simulink model "Dynamic_Wireless_transfer"  (R2024a)
settings: Solver=ode23t  StartTime=0.0  StopTime=10  RelTol=1e-3
undefined symbols (not defined in the file): Ion, Lithium
libraries: spsSeriesRLCBranchLib x6, spsDiodeLib x4, spsIGBTDiodeLib x4, spsCurrentMeasurementLib x3, spsVoltageMeasurementLib x3, spsACVoltageSourceLib x1, spsBatteryLib x1, spsMutualInductanceLib x1, spsPWMGeneratorDCDCLib x1, spsUniversalBridgeLib x1, sps_lib x1
settings Model: Creator=User  LastModifiedBy=User

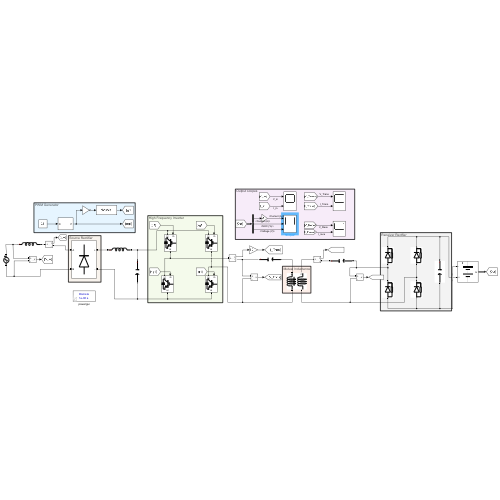
[thumbnail: Simulink's stored preview of the top-level diagram]
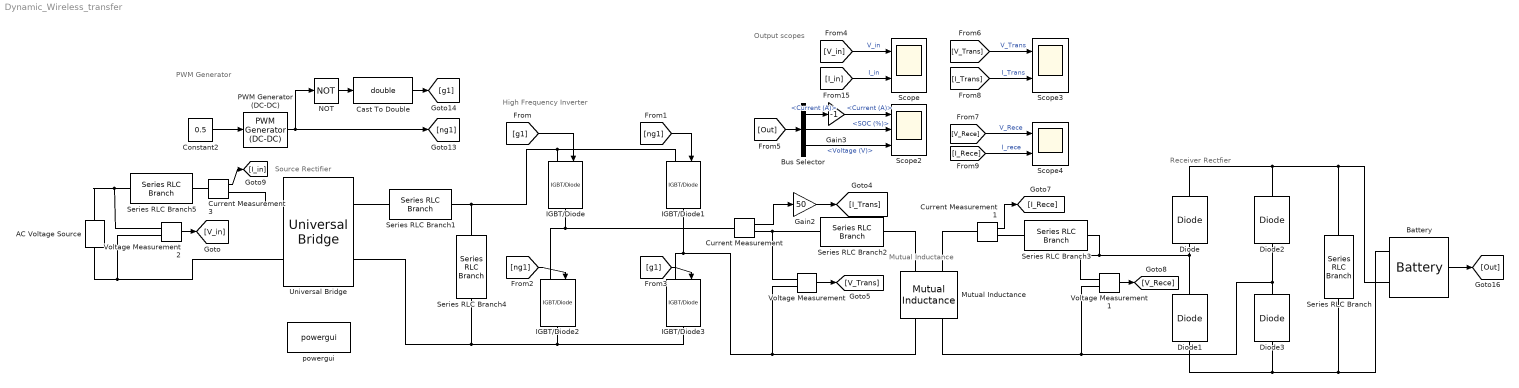
== system Dynamic_Wireless_transfer ==
  note: PWM Generator
  note: Mutual Inductance
  note: Source Rectifier
  note: Output scopes
  note: Receiver Rectfier
  note: High Frequency Inverter
  AC Voltage Source : spsACVoltageSourceLib/AC Voltage Source  Amplitude=500  Phase=180  Frequency=60  SampleTime=0  Measurements=Voltage  BusType=swing  Pref=10e3  Qref=0  Qmin=-inf  Qmax=+inf
  Battery : spsBatteryLib/Battery  BatType=Lithium-Ion  ShowTempParam=off  ThermalPreset=no  ShowAgeParam=off  NomV=360  NomQ=100  SOC=50  Batt_Tr=10  PresetModel=on  MaxQ=100  MinV=270  FullV=419.0354  Dis_rate=43.4783  R=0.036  Normal_OP=90.4348  expZone="[388.9389      4.913043]"  current=[6.5 13 32.5]  Units=Time  Tci=20  NomT=20  T2=-30  MaxQ2=4.8  FullV2=7.1  Normal_OP2=5.655  expZone2="[6.58           1]"  Rca=0.6  ti=2000  Dp=0  Neq0=0  Tsim=1e6  Ta1=25  Qeol=5.4*0.9  Reol=0.013333*1.2  Char_age=[2.3478, 3]  Dis_age=[2.3478, 10]  N1=1500  N2=10500  N3=1000  N4=1400  Ta2=45  N5=950
  Bus Selector : BusSelector  OutputSignals=Current (A),SOC (%),Voltage (V)
  Cast To Double : DataTypeConversion  OutDataTypeStr=double  SaturateOnIntegerOverflow=off  RndMeth=Floor
  Constant2 : Constant  Value=0.5
  Current Measurement : spsCurrentMeasurementLib/Current Measurement  PhasorSimulation=off  OutputType=Complex  PSBequivalent=0
  Current Measurement1 : spsCurrentMeasurementLib/Current Measurement  PhasorSimulation=off  OutputType=Complex  PSBequivalent=0
  Current Measurement3 : spsCurrentMeasurementLib/Current Measurement  PhasorSimulation=off  OutputType=Complex  PSBequivalent=0
  Diode{,1..3} (4 alike) : spsDiodeLib/Diode  Ron=0.001  Lon=0  Vf=0.8  IC=0  UseSnubber=0  Rs=500  Cs=250e-9  Measurements=off
  Gain2 : Gain  Gain=50
  Gain3 : Gain  Gain=-1
  IGBT/Diode{,1..3} (4 alike) : spsIGBTDiodeLib/IGBT//Diode  Ron=1e-3  Rs=1e5  Cs=inf  Measurements=off
  Mutual Inductance : spsMutualInductanceLib/Mutual Inductance  LConnTagsString=a|b  RConnTagsString=A|B  TypeOfMutual=Two or three windings with equal mutual terms  NumberOfWindings=3  SelfImpedance1=[1e-3 266.16e-6]  SelfImpedance2=[1e-3 256.79e-6]  ThreeWindings=off  SelfImpedance3=[ 1.1 1.1e-03]  MutualImpedance=[0 85.46e-6]  InductanceMatrix="[1.0 0.9  0.9 ;  0.9 1.0  0.9;  0.9 0.9 1.0 ] * 1e-3"  ResistanceMatrix="[1.0 0.9  0.9 ;  0.9 1.0  0.9;  0.9 0.9 1.0 ]"  Measurements=None
      settings: LibrarySourceBlock=sps_lib/Passives/Mutual Inductance
  NOT : Logic  Operator=NOT  IconShape=distinctive  AllPortsSameDT=off  OutDataTypeStr=boolean
  PWM Generator (DC-DC) : spsPWMGeneratorDCDCLib/PWM Generator (DC-DC)  Fsw=30000  Ts=0
  Scope : Scope  NumInputPorts=2
  Scope2 : Scope  NumInputPorts=3
  Scope3 : Scope  NumInputPorts=2
  Scope4 : Scope  NumInputPorts=2
  Series RLC Branch : spsSeriesRLCBranchLib/Series RLC Branch  LConnTagsString=__new0  RConnTagsString=__new0  BranchType=C  Resistance=1  Inductance=1e-3  SetiL0=off  InitialCurrent=0  Capacitance=300e-6  Setx0=off  InitialVoltage=0  Measurements=None
  Series RLC Branch1 : spsSeriesRLCBranchLib/Series RLC Branch  LConnTagsString=__new0  RConnTagsString=__new0  BranchType=L  Resistance=1  Inductance=10e-3  SetiL0=off  InitialCurrent=0  Capacitance=1e-8  Setx0=off  InitialVoltage=0  Measurements=None
  Series RLC Branch2 : spsSeriesRLCBranchLib/Series RLC Branch  LConnTagsString=__new0  RConnTagsString=__new0  BranchType=C  Resistance=1  Inductance=1e-3  SetiL0=off  InitialCurrent=0  Capacitance=105.74e-9  Setx0=off  InitialVoltage=0  Measurements=None
  Series RLC Branch3 : spsSeriesRLCBranchLib/Series RLC Branch  LConnTagsString=__new0  RConnTagsString=__new0  BranchType=C  Resistance=1  Inductance=1e-3  SetiL0=off  InitialCurrent=0  Capacitance=109.69e-9  Setx0=off  InitialVoltage=0  Measurements=None
  Series RLC Branch4 : spsSeriesRLCBranchLib/Series RLC Branch  LConnTagsString=__new0  RConnTagsString=__new0  BranchType=C  Resistance=1  Inductance=1e-3  SetiL0=off  InitialCurrent=0  Capacitance=300e-6  Setx0=off  InitialVoltage=0  Measurements=None
  Series RLC Branch5 : spsSeriesRLCBranchLib/Series RLC Branch  LConnTagsString=__new0  RConnTagsString=__new0  BranchType=L  Resistance=1  Inductance=100e-3  SetiL0=off  InitialCurrent=0  Capacitance=1e-6  Setx0=off  InitialVoltage=0  Measurements=None
  Universal Bridge : spsUniversalBridgeLib/Universal Bridge  Arms=2  SnubberResistance=1e5  SnubberCapacitance=inf  Device=Diodes  Ron=1e-3  Lon=0  ForwardVoltages="[  0  0  ]"  ForwardVoltage=0  GTOparameters=[ 10e-6 , 20e-6 ]  IGBTparameters=[ 1e-6 , 2e-6 ]  Measurements=All voltages and currents  Measurements_2=None  converterType=Rectifier
  Voltage Measurement : spsVoltageMeasurementLib/Voltage Measurement  PhasorSimulation=off  OutputType=Complex  PSBequivalent=0
  Voltage Measurement1 : spsVoltageMeasurementLib/Voltage Measurement  PhasorSimulation=off  OutputType=Complex  PSBequivalent=0
  Voltage Measurement2 : spsVoltageMeasurementLib/Voltage Measurement  PhasorSimulation=off  OutputType=Complex  PSBequivalent=0
  powergui : sps_lib/powergui  Priority=1  SimulationMode=Discrete  SampleTime=1e-6  frequency=60  Iterations=50  frequencyindice=0  Pbase=100e6  ErrMax=1e-4  UnitsV=kV  UnitsW=MW  buscounter=0  FunctionMessages=off  echomessages=off  EnableUseOfTLC=off  CurrentSourceSwitches=off  DisableSnubberDevices=off  DisableRonSwitches=off  DisableVfSwitches=off  DisplayEquations=off  AutomaticDiscreteSolvers=off  SolverType=Tustin/Backward Euler (TBE)  Interpol=off  ExternalGateDelay=off  methode=off  Ts=100  x0status=blocks  SPID=on  SwTol=0  HookPort=off  NonlinearTolerance=1e-4  nMaxIteration=100  ContinueOnMaxIteration=off  RestoreLinks=warning  ResistiveCurrentMeasurement=off  Frange=[0:2:500]  Ylog=off  Xlog=on  ShowGrid=off  save=off  variable=ZData  structure=0  ZoomFFT=off  StartTime=0.0  cycles=1  DisplayStyle=1  fundamental=60  FreqAxis=off  MaxFrequency=1000  frequencyindicesteady=1  RmsSteady=1  display=off
  wires:
  [g1] -> IGBT/Diode/1
  [ng1] -> IGBT/Diode1/1
  [ng1] -> IGBT/Diode2/1
  [g1] -> IGBT/Diode3/1
  Current Measurement/1 -> Gain2/1
  Voltage Measurement/1 -> [V_Trans]
  Current Measurement1/1 -> [I_Rece]
  Voltage Measurement1/1 -> [V_Rece]
  Gain2/1 -> [I_Trans]
  Constant2/1 -> PWM Generator (DC-DC)/1
  PWM Generator (DC-DC)/1 -> [ng1], NOT/1
  NOT/1 -> Cast To Double/1
  Cast To Double/1 -> [g1]
  [V_Trans] -> Scope3/1  "V_Trans"
  [V_Rece] -> Scope4/1  "V_Rece"
  [I_Trans] -> Scope3/2  "I_Trans"
  Battery/1 -> [Out]
  [Out] -> Bus Selector/1
  Bus Selector/3 -> Scope2/3  "<Voltage (V)>"
  Current Measurement3/1 -> [I_in]
  [I_in] -> Scope/2  "I_in"
  Bus Selector/2 -> Scope2/2  "<SOC (%)>"
  Bus Selector/1 -> Gain3/1  "<Current (A)>"
  [V_in] -> Scope/1  "V_in"
  [I_Rece] -> Scope4/2  "I_rece"
  Gain3/1 -> Scope2/1  "<Current (A)>"
  Voltage Measurement2/1 -> [V_in]
  connections:
  Voltage Measurement/LConn2 -- IGBT/Diode1/RConn1 -- IGBT/Diode3/LConn1 -- Mutual Inductance/RConn1
  IGBT/Diode/RConn1 -- IGBT/Diode2/LConn1 -- Current Measurement/LConn1
  Diode2/LConn1 -- Mutual Inductance/RConn2 -- Voltage Measurement1/LConn2 -- Diode3/RConn1
  Diode/LConn1 -- Series RLC Branch3/RConn1 -- Voltage Measurement1/LConn1 -- Diode1/RConn1
  Diode3/LConn1 -- Series RLC Branch/RConn1 -- Battery/LConn2 -- Diode1/LConn1
  Series RLC Branch2/RConn1 -- Mutual Inductance/LConn1
  Current Measurement/RConn1 -- Series RLC Branch2/LConn1 -- Voltage Measurement/LConn1
  Current Measurement1/LConn1 -- Mutual Inductance/LConn2
  Current Measurement1/RConn1 -- Series RLC Branch3/LConn1
  IGBT/Diode3/RConn1 -- Universal Bridge/RConn2 -- Series RLC Branch4/RConn1 -- IGBT/Diode2/RConn1
  IGBT/Diode1/LConn1 -- Series RLC Branch1/RConn1 -- Series RLC Branch4/LConn1 -- IGBT/Diode/LConn1
  Diode2/RConn1 -- Series RLC Branch/LConn1 -- Battery/LConn1 -- Diode/RConn1
  AC Voltage Source/LConn1 -- Voltage Measurement2/LConn2 -- Universal Bridge/LConn2
  Series RLC Branch1/LConn1 -- Universal Bridge/RConn1
  Current Measurement3/RConn1 -- Universal Bridge/LConn1
  Current Measurement3/LConn1 -- Series RLC Branch5/RConn1
  Series RLC Branch5/LConn1 -- Voltage Measurement2/LConn1 -- AC Voltage Source/RConn1
